simulink model "sim131025"  (R2024a)
settings: Solver=FixedStepAuto  StartTime=0.0  StopTime=150.0  FixedStep=1e-3  RelTol=1e-3
settings Model: Creator=alexe  LastModifiedBy=alexe

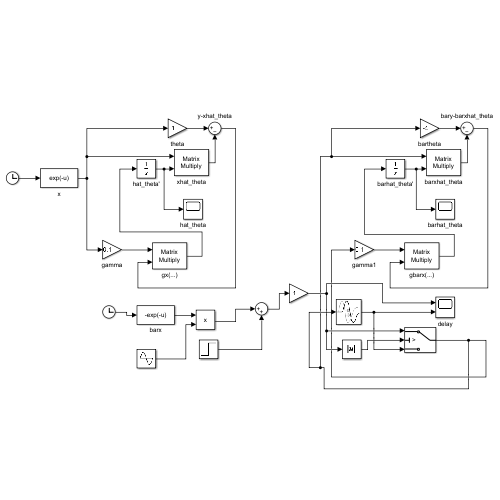
[thumbnail: Simulink's stored preview of the top-level diagram]
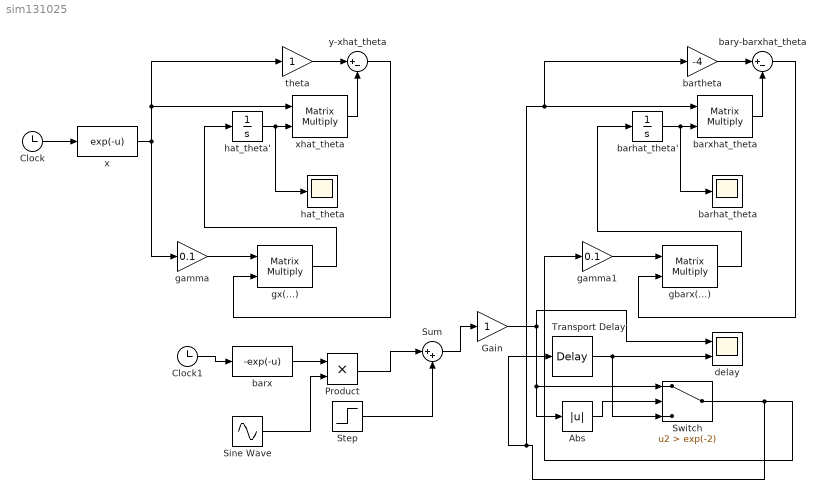
== system sim131025 ==
  Abs : Abs  SaturateOnIntegerOverflow=off
  Clock : Clock
  Clock1 : Clock
  Gain : Gain
  Product : Product
  Sine Wave : Sin  SampleTime=0
  Step : Step  Time=100  SampleTime=0
  Sum : Sum  Inputs=|++
  Switch : Switch  Criteria=u2 > Threshold  Threshold=exp(-2)  SaturateOnIntegerOverflow=off  InputSameDT=off
  Transport Delay : TransportDelay  DelayTime=2
  barhat_theta : Scope
  barhat_theta' : Integrator
  bartheta : Gain  Gain=-4
  barx : Fcn  Expr=-exp(-u)
  barxhat_theta : Product  Multiplication=Matrix(*)
  bary-barxhat_theta : Sum  Inputs=|+-
  delay : Scope  NumInputPorts=2
  gamma : Gain  Gain=0.1
  gamma1 : Gain  Gain=0.1
  gbarx(...) : Product  Multiplication=Matrix(*)
  gx(...) : Product  Multiplication=Matrix(*)
  hat_theta : Scope
  hat_theta' : Integrator
  theta : Gain
  x : Fcn  Expr=exp(-u)
  xhat_theta : Product  Multiplication=Matrix(*)
  y-xhat_theta : Sum  Inputs=|+-
  wires:
  Clock/1 -> x/1
  x/1 -> theta/1, xhat_theta/1, gamma/1
  hat_theta'/1 -> hat_theta/1, xhat_theta/2
  theta/1 -> y-xhat_theta/1
  xhat_theta/1 -> y-xhat_theta/2
  gamma/1 -> gx(...)/1
  y-xhat_theta/1 -> gx(...)/2
  gx(...)/1 -> hat_theta'/1
  barhat_theta'/1 -> barhat_theta/1, barxhat_theta/2
  bartheta/1 -> bary-barxhat_theta/1
  gbarx(...)/1 -> barhat_theta'/1
  bary-barxhat_theta/1 -> gbarx(...)/2
  Clock1/1 -> barx/1
  gamma1/1 -> gbarx(...)/1
  barxhat_theta/1 -> bary-barxhat_theta/2
  Transport Delay/1 -> Switch/3, delay/2
  Switch/1 -> gamma1/1, bartheta/1, barxhat_theta/1, Transport Delay/1
  Gain/1 -> delay/1, Abs/1, Switch/1
  Sum/1 -> Gain/1
  Step/1 -> Sum/2
  Abs/1 -> Switch/2
  barx/1 -> Product/1
  Product/1 -> Sum/1
  Sine Wave/1 -> Product/2
